simulink model "brk_ut"  (Simulink 8.1)
settings: Solver=FixedStepDiscrete  StartTime=0.0  StopTime=Inf  FixedStep=0.005  RelTol=1e-3
libraries: siltestlib x3, brk x1
settings Model: Creator=xsellart  LastModifiedBy=AT015555
settings DataIOCC: SignalLoggingSaveFormat=Dataset
settings OptimizationCC: ExpressionDepthLimit=128
settings DebuggingCC: FcnCallInpInsideContextMsg=EnableAllAsError
settings GRTTargetCC: CombineOutputUpdateFcns=on  GRTInterface=off

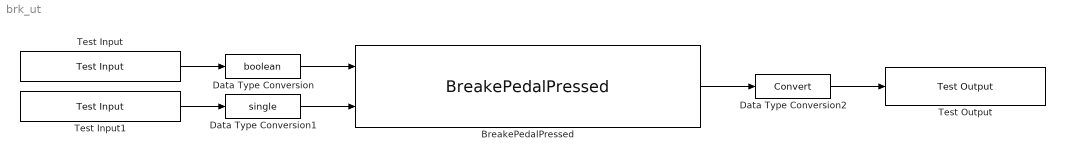
== system brk_ut ==
  BreakePedalPressed : brk/BreakePedalPressed
  Data Type Conversion : DataTypeConversion  OutDataTypeStr=boolean
  Data Type Conversion1 : DataTypeConversion  OutDataTypeStr=single
  Data Type Conversion2 : DataTypeConversion
  Test Input : siltestlib/Test Input  varname=VDINR_DriverBrakPedalOn_flg  sampletime=0.005
  Test Input1 : siltestlib/Test Input  varname=VDINR_MCPressure_bar  sampletime=0.005
  Test Output : siltestlib/Test Output  varname=VIFO_BrakePedalPressed_flg  sampletime=-1
  wires:
  Test Input/1 -> Data Type Conversion/1
  Data Type Conversion/1 -> BreakePedalPressed/1
  Test Input1/1 -> Data Type Conversion1/1
  Data Type Conversion1/1 -> BreakePedalPressed/2
  BreakePedalPressed/1 -> Data Type Conversion2/1
  Data Type Conversion2/1 -> Test Output/1
